simulink model "TST_MRly_VD"  (R2016b)
settings: Solver=FixedStepDiscrete  StartTime=0.0  StopTime=simTime  FixedStep=sampleTime  RelTol=1e-3
values from neighbouring files (symbols this model uses):
  testCase = 1    [initTST_MRly_VD_001.m]
libraries: simulink x4, UnitTest_Lib x2
settings Model: Creator=zhengjinyan  LastModifiedBy=zhengjinyan
settings DebuggingCC: SignalRangeChecking=error

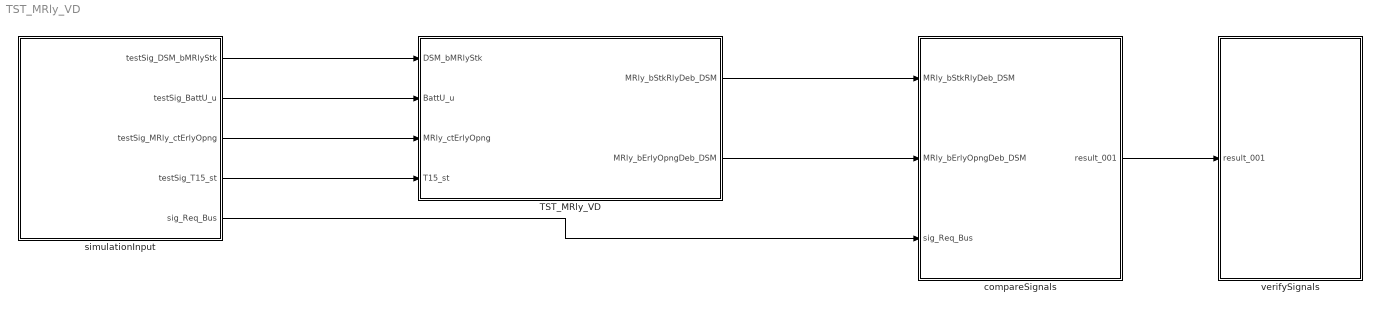
== system TST_MRly_VD ==
  TST_MRly_VD : Subsystem
  compareSignals : Subsystem
  simulationInput : Subsystem
  verifySignals : Subsystem
  wires:
  simulationInput/1(testSig_DSM_bMRlyStk) -> TST_MRly_VD/1(DSM_bMRlyStk)
  simulationInput/2(testSig_BattU_u) -> TST_MRly_VD/2(BattU_u)
  simulationInput/3(testSig_MRly_ctErlyOpng) -> TST_MRly_VD/3(MRly_ctErlyOpng)
  simulationInput/4(testSig_T15_st) -> TST_MRly_VD/4(T15_st)
  TST_MRly_VD/1(MRly_bStkRlyDeb_DSM) -> compareSignals/1(MRly_bStkRlyDeb_DSM)
  TST_MRly_VD/2(MRly_bErlyOpngDeb_DSM) -> compareSignals/2(MRly_bErlyOpngDeb_DSM)
  simulationInput/5(sig_Req_Bus) -> compareSignals/3(sig_Req_Bus)
  compareSignals/1(result_001) -> verifySignals/1(result_001)

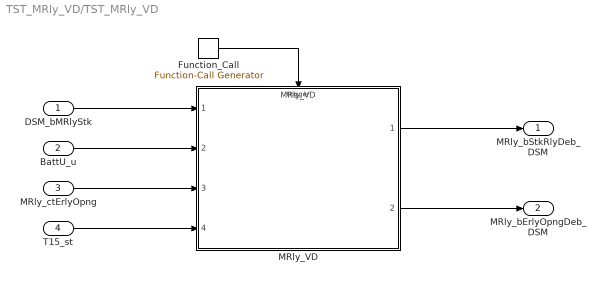
== system TST_MRly_VD/TST_MRly_VD ==
  DSM_bMRlyStk : Inport
  BattU_u : Inport  Port=2
  MRly_ctErlyOpng : Inport  Port=3
  T15_st : Inport  Port=4
  Function_Call : simulink/Ports & Subsystems/Function-Call Generator  sample_time=sampleTime  numberOfIterations=1
  MRly_VD : ModelReference  ModelNameDialog=MRly_VD  SimulationMode=Normal  ModelReferenceVersion=1.16  TriggerPortName=function  TriggerPortTriggerType=function-call  TriggerPortStatesWhenEnabling=held
  MRly_bStkRlyDeb_DSM : Outport
  MRly_bErlyOpngDeb_DSM : Outport  Port=2
  wires:
  Function_Call/1 -> MRly_VD/Trigger
  DSM_bMRlyStk/1 -> MRly_VD/1
  BattU_u/1 -> MRly_VD/2
  MRly_ctErlyOpng/1 -> MRly_VD/3
  T15_st/1 -> MRly_VD/4
  MRly_VD/1 -> MRly_bStkRlyDeb_DSM/1
  MRly_VD/2 -> MRly_bErlyOpngDeb_DSM/1

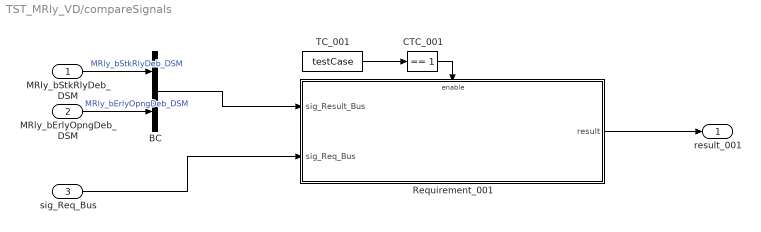
== system TST_MRly_VD/compareSignals ==
  MRly_bStkRlyDeb_DSM : Inport
  MRly_bErlyOpngDeb_DSM : Inport  Port=2
  sig_Req_Bus : Inport  Port=3
  BC : BusCreator  Inputs=2
  CTC_001 : simulink/Logic and Bit Operations/Compare To Constant  relop===  const=1  OutDataTypeStr=boolean
  Requirement_001 : Subsystem
  TC_001 : Constant  Value=testCase
  result_001 : Outport
  wires:
  MRly_bStkRlyDeb_DSM/1 -> BC/1  "MRly_bStkRlyDeb_DSM"
  MRly_bErlyOpngDeb_DSM/1 -> BC/2  "MRly_bErlyOpngDeb_DSM"
  TC_001/1 -> CTC_001/1
  CTC_001/1 -> Requirement_001/Enable
  sig_Req_Bus/1 -> Requirement_001/2(sig_Req_Bus)
  BC/1 -> Requirement_001/1(sig_Result_Bus)
  Requirement_001/1(result) -> result_001/1

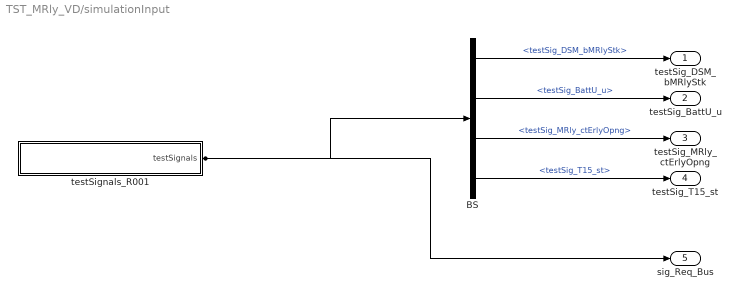
== system TST_MRly_VD/simulationInput ==
  BS : BusSelector  OutputSignals=testSig_DSM_bMRlyStk,testSig_BattU_u,testSig_MRly_ctErlyOpng,testSig_T15_st
  testSignals_R001 : Subsystem
  testSig_DSM_bMRlyStk : Outport
  testSig_BattU_u : Outport  Port=2
  testSig_MRly_ctErlyOpng : Outport  Port=3
  testSig_T15_st : Outport  Port=4
  sig_Req_Bus : Outport  Port=5
  wires:
  BS/1 -> testSig_DSM_bMRlyStk/1  "<testSig_DSM_bMRlyStk>"
  BS/2 -> testSig_BattU_u/1  "<testSig_BattU_u>"
  BS/3 -> testSig_MRly_ctErlyOpng/1  "<testSig_MRly_ctErlyOpng>"
  BS/4 -> testSig_T15_st/1  "<testSig_T15_st>"
  testSignals_R001/1(testSignals) -> BS/1, sig_Req_Bus/1

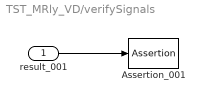
== system TST_MRly_VD/verifySignals ==
  result_001 : Inport
  Assertion_001 : Assertion  Enabled=off
  wires:
  result_001/1 -> Assertion_001/1

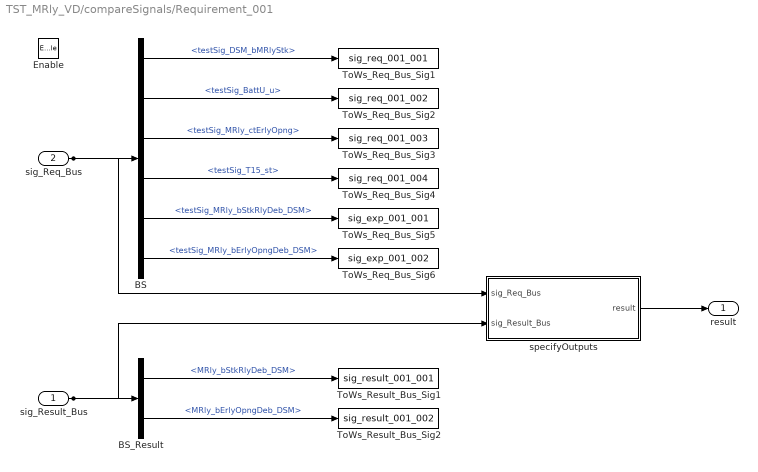
== system TST_MRly_VD/compareSignals/Requirement_001 ==
  sig_Result_Bus : Inport
  sig_Req_Bus : Inport  Port=2
  Enable : EnablePort
  BS : BusSelector  OutputSignals=testSig_DSM_bMRlyStk,testSig_BattU_u,testSig_MRly_ctErlyOpng,testSig_T15_st,testSig_MRly_bStkRlyDeb_DSM,testSig_MRly_bErlyOpngDeb_DSM
  BS_Result : BusSelector  OutputSignals=MRly_bStkRlyDeb_DSM,MRly_bErlyOpngDeb_DSM
  ToWs_Req_Bus_Sig1 : ToWorkspace  VariableName=sig_req_001_001  SaveFormat=Structure With Time
  ToWs_Req_Bus_Sig2 : ToWorkspace  VariableName=sig_req_001_002  SaveFormat=Structure With Time
  ToWs_Req_Bus_Sig3 : ToWorkspace  VariableName=sig_req_001_003  SaveFormat=Structure With Time
  ToWs_Req_Bus_Sig4 : ToWorkspace  VariableName=sig_req_001_004  SaveFormat=Structure With Time
  ToWs_Req_Bus_Sig5 : ToWorkspace  VariableName=sig_exp_001_001  SaveFormat=Structure With Time
  ToWs_Req_Bus_Sig6 : ToWorkspace  VariableName=sig_exp_001_002  SaveFormat=Structure With Time
  ToWs_Result_Bus_Sig1 : ToWorkspace  VariableName=sig_result_001_001  SaveFormat=Structure With Time
  ToWs_Result_Bus_Sig2 : ToWorkspace  VariableName=sig_result_001_002  SaveFormat=Structure With Time
  specifyOutputs : Subsystem
  result : Outport
  wires:
  sig_Req_Bus/1 -> BS/1, specifyOutputs/1(sig_Req_Bus)
  BS/1 -> ToWs_Req_Bus_Sig1/1  "<testSig_DSM_bMRlyStk>"
  BS/2 -> ToWs_Req_Bus_Sig2/1  "<testSig_BattU_u>"
  BS/3 -> ToWs_Req_Bus_Sig3/1  "<testSig_MRly_ctErlyOpng>"
  BS/4 -> ToWs_Req_Bus_Sig4/1  "<testSig_T15_st>"
  BS/5 -> ToWs_Req_Bus_Sig5/1  "<testSig_MRly_bStkRlyDeb_DSM>"
  BS/6 -> ToWs_Req_Bus_Sig6/1  "<testSig_MRly_bErlyOpngDeb_DSM>"
  sig_Result_Bus/1 -> BS_Result/1, specifyOutputs/2(sig_Result_Bus)
  BS_Result/1 -> ToWs_Result_Bus_Sig1/1  "<MRly_bStkRlyDeb_DSM>"
  BS_Result/2 -> ToWs_Result_Bus_Sig2/1  "<MRly_bErlyOpngDeb_DSM>"
  specifyOutputs/1(result) -> result/1

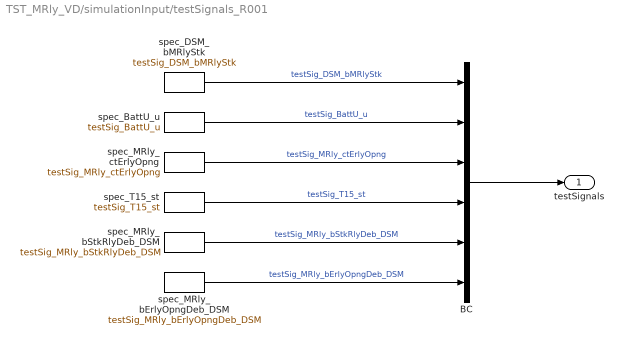
== system TST_MRly_VD/simulationInput/testSignals_R001 ==
  BC : BusCreator  Inputs=6
  spec_BattU_u : FromWorkspace  VariableName=testSig_BattU_u  Interpolate=off  OutputAfterFinalValue=Holding final value
  spec_DSM_bMRlyStk : FromWorkspace  VariableName=testSig_DSM_bMRlyStk  Interpolate=off  OutputAfterFinalValue=Holding final value
  spec_MRly_bErlyOpngDeb_DSM : FromWorkspace  VariableName=testSig_MRly_bErlyOpngDeb_DSM  Interpolate=off  OutputAfterFinalValue=Holding final value
  spec_MRly_bStkRlyDeb_DSM : FromWorkspace  VariableName=testSig_MRly_bStkRlyDeb_DSM  Interpolate=off  OutputAfterFinalValue=Holding final value
  spec_MRly_ctErlyOpng : FromWorkspace  VariableName=testSig_MRly_ctErlyOpng  Interpolate=off  OutputAfterFinalValue=Holding final value
  spec_T15_st : FromWorkspace  VariableName=testSig_T15_st  Interpolate=off  OutputAfterFinalValue=Holding final value
  testSignals : Outport
  wires:
  BC/1 -> testSignals/1
  spec_DSM_bMRlyStk/1 -> BC/1  "testSig_DSM_bMRlyStk"
  spec_BattU_u/1 -> BC/2  "testSig_BattU_u"
  spec_MRly_ctErlyOpng/1 -> BC/3  "testSig_MRly_ctErlyOpng"
  spec_T15_st/1 -> BC/4  "testSig_T15_st"
  spec_MRly_bStkRlyDeb_DSM/1 -> BC/5  "testSig_MRly_bStkRlyDeb_DSM"
  spec_MRly_bErlyOpngDeb_DSM/1 -> BC/6  "testSig_MRly_bErlyOpngDeb_DSM"

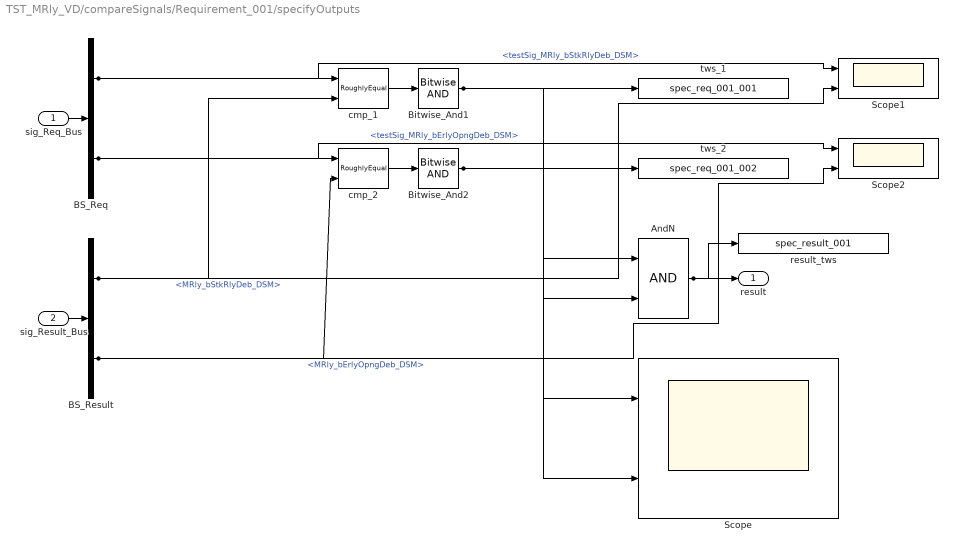
== system TST_MRly_VD/compareSignals/Requirement_001/specifyOutputs ==
  sig_Req_Bus : Inport
  sig_Result_Bus : Inport  Port=2
  AndN : Logic
  BS_Req : BusSelector  OutputSignals=testSig_MRly_bStkRlyDeb_DSM,testSig_MRly_bErlyOpngDeb_DSM
  BS_Result : BusSelector  OutputSignals=MRly_bStkRlyDeb_DSM,MRly_bErlyOpngDeb_DSM
  Bitwise_And1 : simulink/Logic and Bit Operations/Bitwise Operator  logicop=AND  UseBitMask=off  BitMask=bin2dec('11011001')  BitMaskRealWorld=Stored Integer
  Bitwise_And2 : simulink/Logic and Bit Operations/Bitwise Operator  logicop=AND  UseBitMask=off  BitMask=bin2dec('11011001')  BitMaskRealWorld=Stored Integer
  Scope : Scope  NumInputPorts=2
  Scope1 : Scope  NumInputPorts=2
  Scope2 : Scope  NumInputPorts=2
  cmp_1 : UnitTest_Lib/RoughlyEqual  slope=0.1
  cmp_2 : UnitTest_Lib/RoughlyEqual  slope=0.1
  result_tws : ToWorkspace  VariableName=spec_result_001
  tws_1 : ToWorkspace  VariableName=spec_req_001_001
  tws_2 : ToWorkspace  VariableName=spec_req_001_002
  result : Outport
  wires:
  sig_Req_Bus/1 -> BS_Req/1
  sig_Result_Bus/1 -> BS_Result/1
  AndN/1 -> result/1, result_tws/1
  BS_Req/1 -> cmp_1/1, Scope1/1  "<testSig_MRly_bStkRlyDeb_DSM>"
  BS_Result/1 -> cmp_1/2, Scope1/2  "<MRly_bStkRlyDeb_DSM>"
  cmp_1/1 -> Bitwise_And1/1
  Bitwise_And1/1 -> tws_1/1, AndN/1, Scope/1
  BS_Req/2 -> cmp_2/1, Scope2/1  "<testSig_MRly_bErlyOpngDeb_DSM>"
  BS_Result/2 -> cmp_2/2, Scope2/2  "<MRly_bErlyOpngDeb_DSM>"
  cmp_2/1 -> Bitwise_And2/1
  Bitwise_And2/1 -> tws_2/1, AndN/2, Scope/2
